simulink model "system_simulation_tacking_ball"  (R2024a)
settings: Solver=VariableStepAuto  StartTime=0.0  StopTime=2  MaxStep=1e-3  RelTol=1e-3
undefined symbols (not defined in the file or in its folder): A, B, C, F, FI, L, ref
settings Model: Creator=kasper  LastModifiedBy=balder
settings RTWCC: GPUComputeCapability=3.5

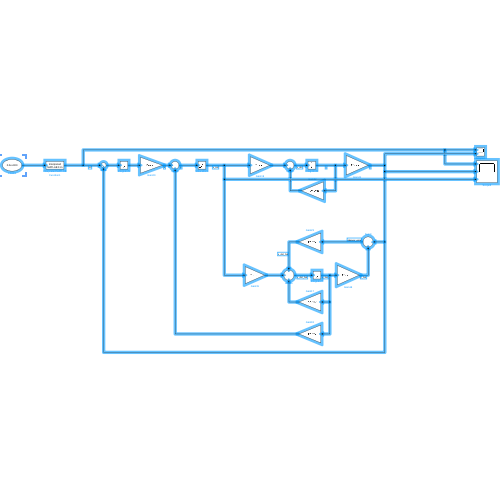
[thumbnail: Simulink's stored preview of the top-level diagram]
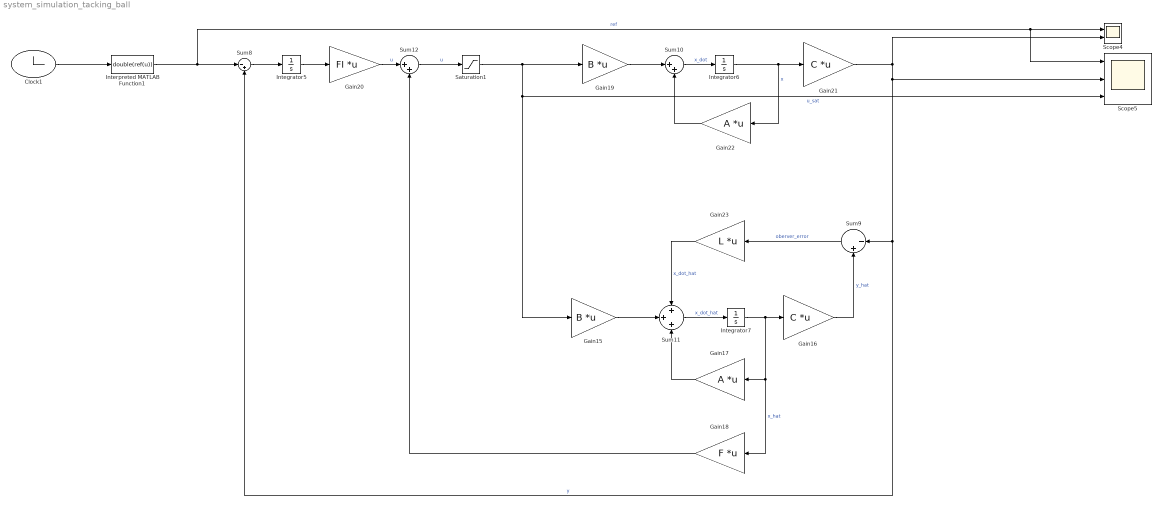
== system system_simulation_tacking_ball ==
  Clock1 : Clock
  Gain15 : Gain  Gain=B  Multiplication=Matrix(K*u) (u vector)
  Gain16 : Gain  Gain=C  Multiplication=Matrix(K*u) (u vector)
  Gain17 : Gain  Gain=A  Multiplication=Matrix(K*u) (u vector)
  Gain18 : Gain  Gain=F  Multiplication=Matrix(K*u) (u vector)
  Gain19 : Gain  Gain=B  Multiplication=Matrix(K*u) (u vector)
  Gain20 : Gain  Gain=FI  Multiplication=Matrix(K*u) (u vector)
  Gain21 : Gain  Gain=C  Multiplication=Matrix(K*u) (u vector)
  Gain22 : Gain  Gain=A  Multiplication=Matrix(K*u) (u vector)
  Gain23 : Gain  Gain=L  Multiplication=Matrix(K*u) (u vector)
  Integrator5 : Integrator
  Integrator6 : Integrator  InitialCondition=zeros(4, 1)
  Integrator7 : Integrator  UpperSaturationLimit=100  LowerSaturationLimit=-100
  Interpreted MATLAB Function1 : MATLABFcn  MATLABFcn=double(ref(u))  Output1D=off
  Saturation1 : Saturate  UpperLimit=12  LowerLimit=-12
  Scope4 : Scope  NumInputPorts=2
  Scope5 : Scope  NumInputPorts=3
  Sum10 : Sum  Inputs=|++
  Sum11 : Sum  Inputs=+++
  Sum12 : Sum  Inputs=|++
  Sum8 : Sum  Inputs=|-+
  Sum9 : Sum  Inputs=|-+
  wires:
  Gain15/1 -> Sum11/2
  Integrator7/1 -> Gain16/1, Gain18/1, Gain17/1  "x_hat"
  Sum9/1 -> Gain23/1  "oberver_error"
  Sum8/1 -> Integrator5/1
  Gain21/1 -> Sum9/1, Sum8/2, Scope5/2, Scope4/2  "y"
  Interpreted MATLAB Function1/1 -> Scope4/1, Scope5/1, Sum8/1  "ref"
  Integrator6/1 -> Gain22/1, Gain21/1  "x"
  Gain18/1 -> Sum12/2
  Clock1/1 -> Interpreted MATLAB Function1/1
  Sum11/1 -> Integrator7/1  "x_dot_hat"
  Sum10/1 -> Integrator6/1  "x_dot"
  Integrator5/1 -> Gain20/1
  Gain16/1 -> Sum9/2  "y_hat"
  Gain23/1 -> Sum11/1  "x_dot_hat"
  Gain19/1 -> Sum10/1
  Gain17/1 -> Sum11/3
  Saturation1/1 -> Gain19/1, Scope5/3, Gain15/1  "u_sat"
  Gain20/1 -> Sum12/1  "u"
  Sum12/1 -> Saturation1/1  "u"
  Gain22/1 -> Sum10/2
